simulink subsystem "actual_discrete_smc_controller"  (R2025a)
settings: Solver=VariableStepAuto  StartTime=0.0  StopTime=10.0  RelTol=1e-3
settings Model: Creator=johnpye  LastModifiedBy=johnpye

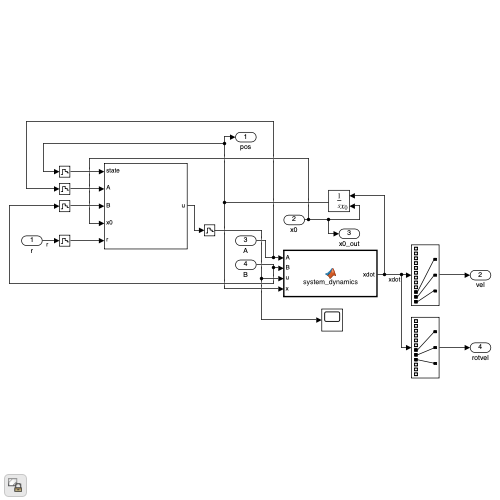
[thumbnail: Simulink's stored preview of the top-level diagram]
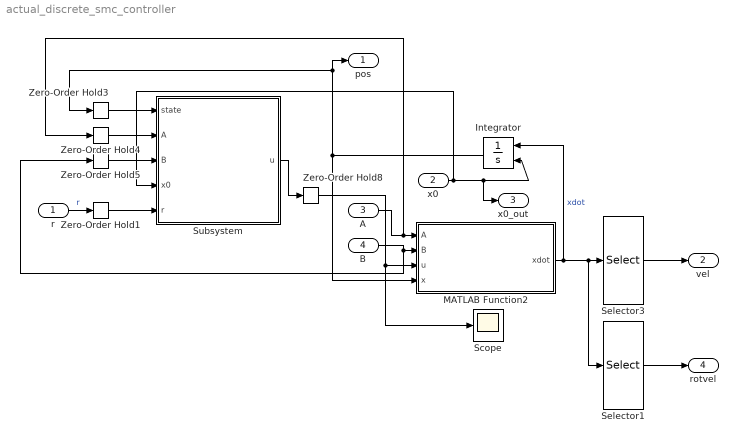
== system actual_discrete_smc_controller ==
  r : Inport
  x0 : Inport  Port=2
  A : Inport  Port=3
  B : Inport  Port=4
  Integrator : Integrator  InitialConditionSource=external
  MATLAB Function2 : MATLAB Function  TreatAsAtomicUnit=on
  Scope : Scope
      settings: ActiveDisplayYMinimum=-14.831202203593328  ActiveDisplayYMaximum=20.695169146470946  DataLoggingVariableName=ScopeData8
  Selector1 : Selector  InputPortWidth=12  IndexOptions=Index vector (dialog)  Indices=[7 8 9]  OutputSizes=1
  Selector3 : Selector  InputPortWidth=12  IndexOptions=Index vector (dialog)  Indices=[10 11 12]  OutputSizes=1
  Subsystem : Subsystem
  Zero-Order Hold{1,3..5,8} (5 alike) : ZeroOrderHold  SampleTime=1/50
  pos : Outport
  vel : Outport  Port=2
  x0_out : Outport  Port=3
  rotvel : Outport  Port=4
  wires:
  Selector3/1 -> vel/1
  x0/1 -> Integrator/2, x0_out/1, Subsystem/4(x0)
  A/1 -> MATLAB Function2/1(A), Zero-Order Hold4/1
  Integrator/1 -> MATLAB Function2/4(x), pos/1, Zero-Order Hold3/1
  B/1 -> Zero-Order Hold5/1, MATLAB Function2/2(B)
  MATLAB Function2/1(xdot) -> Integrator/1, Selector3/1, Selector1/1  "xdot"
  Subsystem/1(u) -> Zero-Order Hold8/1
  Zero-Order Hold1/1 -> Subsystem/5(r)
  Zero-Order Hold3/1 -> Subsystem/1(state)
  Zero-Order Hold4/1 -> Subsystem/2(A)
  Zero-Order Hold5/1 -> Subsystem/3(B)
  Zero-Order Hold8/1 -> MATLAB Function2/3(u), Scope/1
  r/1 -> Zero-Order Hold1/1  "r"
  Selector1/1 -> rotvel/1

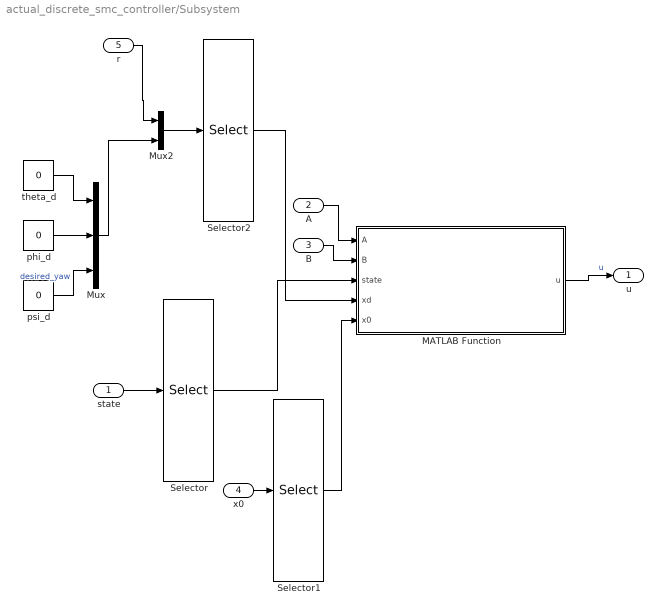
== system actual_discrete_smc_controller/Subsystem ==
  state : Inport
  A : Inport  Port=2
  B : Inport  Port=3
  x0 : Inport  Port=4
  r : Inport  Port=5
  MATLAB Function : MATLAB Function  TreatAsAtomicUnit=on
  Mux : Mux  Inputs=3
  Mux2 : Mux  Inputs=2
  Selector : Selector  InputPortWidth=12  IndexOptions=Index vector (dialog)  Indices=[10 11 12 8 7 9 ]  OutputSizes=1
  Selector1 : Selector  InputPortWidth=12  IndexOptions=Index vector (dialog)  Indices=[10 11 12 8 7 9 ]  OutputSizes=1
  Selector2 : Selector  InputPortWidth=6  IndexOptions=Index vector (dialog)  Indices=[1 2 3 5 4 6]  OutputSizes=1
  phi_d : Constant  Value=0
  psi_d : Constant  Value=0
  theta_d : Constant  Value=0
  u : Outport
  wires:
  Selector2/1 -> MATLAB Function/4(xd)
  Selector1/1 -> MATLAB Function/5(x0)
  Selector/1 -> MATLAB Function/3(state)
  state/1 -> Selector/1
  theta_d/1 -> Mux/1
  x0/1 -> Selector1/1
  Mux2/1 -> Selector2/1
  r/1 -> Mux2/1
  psi_d/1 -> Mux/3  "desired_yaw"
  B/1 -> MATLAB Function/2(B)
  Mux/1 -> Mux2/2
  phi_d/1 -> Mux/2
  A/1 -> MATLAB Function/1(A)
  MATLAB Function/1(u) -> u/1  "u"

== matlab function actual_discrete_smc_controller/MATLAB Function2 ==
  data: A input; B input; u input; x input; xdot output
function xdot = system_dynamics(A, B, u, x)

g = 9.81; % m/s^2
l = 0.2; % m
Jmp = 1e-5; % kgm^2
Jxx = 1.8e-3; % kgm^2
Jyy = 1.8e-3; % kgm^2
Jzz = 1.5e-3; % kgm^2
kmt = 0.1; % m
kwt = 0.1;

K = B(4,2)*Jxx;
m = (1/B(3,1)) * -K;

u = reshape(u, [4, 1]);
x = reshape(x, [12, 1]);
% xdot = A*x + B*u;
xdot=zeros(12,1);

vx = x(1);
vy = x(2);
vz = x(3);
wx = x(4);
wy = x(5);
wz = x(6);
theta = x(7);
phi = x(8);
psi = x(9);
% T = K*u(1);
% Mx = K*u(2);
% My = K*u(3);
% Mz = K*u(4);
T = u(1);
Mx = u(2);
My = u(3);
Mz = u(4);

% Step 3: Calculate derivatives
xdot(1)         = -vz*wy + vy*wz - g*sin(theta);
xdot(2)         = -vx*wz + vz*wx + g*cos(theta)*sin(phi);
xdot(3)         = -vy*wx + vx*wy + g*cos(theta)*cos(phi) - T/m;
xdot(4)         = (1/Jxx)*(-wy*wz*(Jzz - Jyy) + Mx - (kwt/kmt)*Jmp*Mz*wy);
xdot(5)         = (1/Jyy)*(-wx*wz*(Jxx - Jzz) + My - (kwt/kmt)*Jmp*Mz*wx);
xdot(6)         = Mz / Jzz;
xdot(7)         = wy*cos(phi) - wz*sin(phi);
xdot(8)         = wx + wy*sin(phi)*tan(theta) + wz*cos(phi)*tan(theta);
xdot(9)         = wy*(sin(phi)/cos(theta)) + wz*(cos(phi)/cos(theta));
xdot(10)        = vx*cos(psi)*cos(theta) + ...
                    vy*(-sin(psi)*cos(phi) + cos(psi)*sin(theta)*sin(phi)) + ...
                    vz*(sin(psi)*sin(phi) + cos(psi)*sin(theta)*cos(phi));
xdot(11)        = vx*sin(psi)*cos(theta) + ...
                    vy*(cos(psi)*cos(phi) + sin(psi)*sin(theta)*sin(phi)) + ...
                    vz*(-cos(psi)*sin(phi) + sin(psi)*sin(theta)*cos(phi));
xdot(12)        = vx*sin(theta) - vy*cos(theta)*sin(phi) - vz*cos(theta)*cos(phi);

== matlab function actual_discrete_smc_controller/Subsystem/MATLAB Function ==
  data: A input; B input; state input; u output; xd input size=[6; 1]; x0 input
function u = MATLAB_Function(A, B, state, xd, x0)
persistent xk;
persistent xkp1;
persistent xk_d;
persistent xkp1_d;
persistent ukm1;

% xd(2) = -xd(2);
% xd(3) = -xd(3);

if isempty(xk)
    xk = x0;
    xkp1 = xk;
    xk_d = xd;
    xkp1_d = xd;
    ukm1 = zeros(4,1);
end

if abs(norm(xkp1 - state)) > 1e-9
    xk = xkp1;
    xkp1 = state;
end
if abs(norm(xkp1_d - xk_d)) > 1e-9
    xk_d = xkp1_d;
    xkp1_d = xd;
end
if abs(norm(xkp1_d - xd)) > 1e-9
    xk_d = xkp1_d;
    xkp1_d = xd;
end

% g = 9.81; % m/s^2
% l = 0.2; % m
% m = 0.8; % kg
% Jmp = 0;
% Jxx = 1.8e-3; % kgm^2
% Jyy = 1.8e-3; % kgm^2
% Jzz = 1.5e-3; % kgm^2
% kmt = 0.1; % m
dt = 1/50;
g = 9.81;
m = 0.8;
Jxx = 1.8e-3; % kgm^2
Jyy = 1.8e-3; % kgm^2
Jzz = 1.5e-3; % kgm^2
l = 0.2; % m
Jmp = 1e-5; % kgm^2
K1 = 0.0001;
K2 = 0.0001;
K3 = 0.0001;
K4 = 0.0012;
K5 = 0.0012;
K6 = 0.0012;
nuz = 7;
nupsi = 7; 
nu3 = 14;
nu4 = 14;
az = 6;
apsi = 1;
b = 5;
d = 2;
TM = [b b b b;
      0 -b 0 b;
      -b 0 b 0;
      d -d d -d];
Omegas = inv(TM)*ukm1;
Omegas = real(sqrt(complex(Omegas)));
Omegar = real(Omegas(1) - Omegas(2) + Omegas(3) - Omegas(4));

u = zeros(4,1);

dxk   = (xkp1 - xk)/dt;
dxk_d = (xkp1_d - xk_d)/dt; % should be zero

szk = az*(xk_d(3) - xk(3)) + (dxk_d(3) - dxk(3));
szk = min(szk, 2);
szk = max(szk, -2);
spsik = apsi*(xk_d(6) - xk(6)) + (dxk_d(6) - dxk(6));
spsik = min(spsik, 2);
spsik = max(spsik, -2);

u_T = (m/(cos(xk(4))*cos(xk(5))))*(-az*dxk(3) + (K3/m)*dxk(3) + g + nuz*szk);
u_Mz = Jzz*(( -apsi*dxk(6) + (K6/Jzz)*dxk(6) ) + nupsi*spsik);

a1 = 6*m/(u_T*cos(xk(6))); % 6
a2 = 2*m/(u_T*cos(xk(6))); % 2
a3 = 2; 
a4 = 8; 
a5 = -6*m/(u_T*cos(xk(4))*cos(xk(6))); % 6
a6 = -2*m/(u_T*cos(xk(4))*cos(xk(6))); % 2
a7 = 2; 
a8 = 8; %

sphik = a1*(dxk_d(2) - dxk(2)) + a2*(xk_d(2) - xk(2)) + a3*(dxk_d(4) - dxk(4)) + a4*(xk_d(4) - xk(4));
% sphik = min(sphik, 4);
% sphik = max(sphik, -4);
sthetak = a5*(dxk_d(1) - dxk(1)) + a6*(xk_d(1) - xk(1)) + a7*(dxk_d(5) - dxk(5)) + a8*(xk_d(5) - xk(5));
% sthetak = min(sthetak, 4);
% sthetak = max(sthetak, -4);

g1_k = (cos(xk(4))*sin(xk(5))*sin(xk(6)) - sin(xk(4))*cos(xk(6)))/m;
g2_k = (cos(xk(4))*sin(xk(5))*cos(xk(6)) + sin(xk(4))*sin(xk(6)))/m;
f1_k = ( dxk(5)*dxk(6)*(Jyy - Jzz) + Jmp*dxk(5)*Omegar - K4*l*dxk(4) )/Jxx;
f2_k = ( dxk(6)*dxk(4)*(Jzz - Jxx) - Jmp*dxk(4)*Omegar - K5*l*dxk(5) )/Jyy;

u_Mx = (Jxx/(l*a3))*(-a1*(g1_k*u_T - (K2*dxk(2)/m)) - a2*dxk(2) - a3*f1_k - a4*dxk(4) + nu3*sphik);
u_My = (Jyy/(l*a7))*(-a5*(g2_k*u_T - (K1*dxk(1)/m)) - a6*dxk(1) - a7*f2_k - a8*dxk(5) + nu4*sthetak);

u(1) = u_T;
u(2) = u_Mx;
u(3) = u_My;
u(4) = u_Mz;
ukm1 = u;
